simulink model "lqi"  (R2023b)
settings: Solver=VariableStepAuto  StartTime=0.0  StopTime=10.0  RelTol=1e-3
settings Model: Creator=Matthew  LastModifiedBy=Matthew

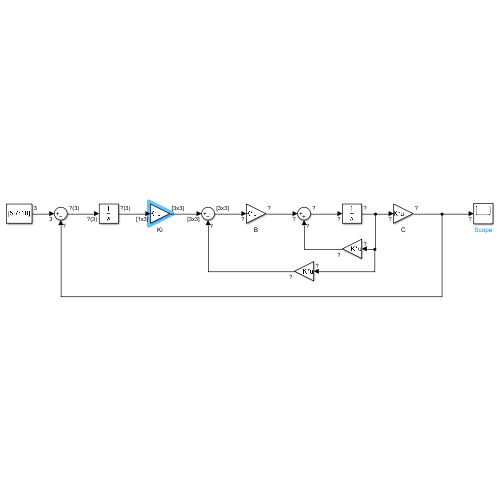
[thumbnail: Simulink's stored preview of the top-level diagram]
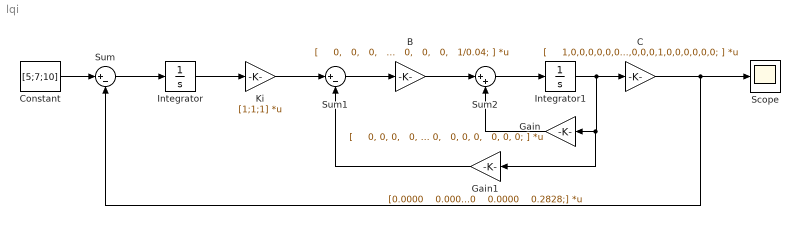
== system lqi ==
  B : Gain  Gain=|  Multiplication=Matrix(K*u)
      | [
      |     0,   0,   0,   0;
      |     0,   0,   0,   0;
      |     0,   0,   0,   0;
      |     
      |     0,   0,   0,   0;
      |     0,   0,   0,   0;
      |     0,   0,   0,   0;
      |     
      |     0,   0,   0,   0;
      |     0,   0,   0,   0;
      |     1/1,  0,   0,   0;
      |     
      |     0,   1/0.11, 0,   0;
      |     0,   0,   1/0.11, 0;
      |     0,   0,   0,   1/0.04;
      | ]
  C : Gain  Gain=|  Multiplication=Matrix(K*u)
      | [
      |     1,0,0,0,0,0,0,0,0,0,0,0;
      |     0,1,0,0,0,0,0,0,0,0,0,0;
      |     0,0,1,0,0,0,0,0,0,0,0,0;
      |     0,0,0,1,0,0,0,0,0,0,0,0;
      |     0,0,0,0,1,0,0,0,0,0,0,0;
      |     0,0,0,0,0,1,0,0,0,0,0,0;
      | ]
  Constant : Constant  Value=[5;7;10]
  Gain : Gain  Gain=|  Multiplication=Matrix(K*u)
      | [
      |     0, 0, 0,   0, 0, 0,   1, 0, 0,   0, 0, 0;
      |     0, 0, 0,   0, 0, 0,   0, 1, 0,   0, 0, 0;
      |     0, 0, 0,   0, 0, 0,   0, 0, 1,   0, 0, 0;
      |     
      |     0, 0, 0,   0, 0, 0,   0, 0, 0,   1, 0, 0;
      |     0, 0, 0,   0, 0, 0,   0, 0, 0,   0, 1, 0;
      |     0, 0, 0,   0, 0, 0,   0, 0, 0,   0, 0, 1;
      | 
      |     0, 0, 0,   0, 9.81, 0,   0, 0, 0,   0, 0, 0;
      |     0, 0, 0,   -9.81,0, 0,   0, 0, 0,   0, 0, 0;
      |     0, 0, 0,   0, 0, 0,   0, 0, 0,   0, 0, 0;
      | 
      |     0, 0, 0,   0, 0, 0,   0, 0, 0,   0, 0, 0;
      |     0, 0, 0,   0, 0, 0,   0, 0, 0,   0, 0, 0;
      |     0, 0, 0,   0, 0, 0,   0, 0, 0,   0, 0, 0;
      | ]
  Gain1 : Gain  Gain=|  Multiplication=Matrix(K*u)
      | [0.0000    0.0000    1.0000   -0.0000    0.0000    0.0000    0.0000    0.0000    1.4142   -0.0000    0.0000   -0.0000;
      |     0.0000   -1.0000   -0.0000    3.8547    0.0000    0.0000    0.0000   -0.8865   -0.0000    0.9209    0.0000    0.0000;
      |     1.0000    0.0000    0.0000   -0.0000    3.8547    0.0000    0.8865    0.0000   -0.0000    0.0000    0.9209    0.0000;
      |     0.0000    0.0000    0.0000   -0.0000    0.0000    1.0000   -0.0000    0.0000   -0.0000   -0.0000    0.0000    0.2828;]
  Integrator : Integrator
  Integrator1 : Integrator
  Ki : Gain  Gain=[1;1;1]  Multiplication=Matrix(K*u)
  Scope : Scope
  Sum : Sum  Inputs=|+-
  Sum1 : Sum  Inputs=|+-
  Sum2 : Sum  Inputs=|++
  wires:
  Constant/1 -> Sum/1
  Sum/1 -> Integrator/1
  Integrator/1 -> Ki/1
  Ki/1 -> Sum1/1
  Sum1/1 -> B/1
  B/1 -> Sum2/1
  Sum2/1 -> Integrator1/1
  Gain/1 -> Sum2/2
  Integrator1/1 -> Gain1/1, Gain/1, C/1
  C/1 -> Sum/2, Scope/1
  Gain1/1 -> Sum1/2
